simulink model "processor_with_peripherals"  (R2025a)
settings: Solver=FixedStepDiscrete  StartTime=0.0  StopTime=inf  RelTol=1e-3
libraries: simulink x6
(part 2 of 5)

== system processor_with_peripherals/Processor ==
  In1 : Inport
  Common hardware : Subsystem
  Core_0 : Subsystem
  Core_1 : Subsystem
  Core_2 : Subsystem
  Core_3 : Subsystem
  Instruction_Memory_{0..3} (4 alike) : LookupNDDirect  NumberOfTableDimensions=1  Table=[808464698;808464432;926496560;1144140337;1144402484;1145123890;1128608816;1144401989;1127362614;892810038;221463092;808532490;808529968;808464432;892874808;959460404;959985974;858798390;876098866;825771568;1144469044;1162098229;825887245;842018864;909127728;1110454339;909193785;960639283;825241653;943009843;842023737;826356273;859125811;973737267;808464433;808464435;843266352;1093810480;926167618;925906232;910378291;892351281;1160982584;808470085;168637495;808464698;808465456;909130032;1111049269;926496582;1144140337;1144402484;1145123890;1128608816;1144401989;221852470;808532490;808792112;926101552;808466741;892874808;959985972;959460406;858797110;959984946;1144473136;893662773;825887245;909127728;909127728;925904963;1160983097;859975987;826689077;943011891;1160921908;825766449;892678195;973737271;808464433;808464439;843265072;942815555;927089732;825307444;909390128;892612921;892614962;910374448;168641336;808464698;808466480;842610480;892813878;942682167;1093874224;808927555;1128542533;909719609;875640885;221458999;808532490;809054256;959459376;825767732;858863156;808465968;859385905;892613944;858862659;808465712;927281200;825887245;1093677104;1160785968;1144008774;943140912;943011385;808924209;943141941;825635889;808857651;959459632;973737272;808464433;808464450;892875577;893596976;892351281;875573300;808470085;909127733;808470085;926036034;168638278;808464698;808469296;1093742640;926103344;859058224;1093742640;926103344;859058224;1093742640;808927792;221328951;808532490;809775152;842018864;1127821364;825504564;892350769;1160984372;843200067;927086388;842020656;875966516;825887245;1160785968;959459376;876036920;942747697;909129778;808662323;825372725;1177892659;1095118901;859255876;973737264;808464433;808464454;1160852278;808465734;925906754;808727088;859063097;860041529;1178745155;925906754;168636721;808464698;808464433;875638832;876099888;876823607;909325875;808928819;1094267696;942815288;808923952;221398071;808532490;808530224;825241648;858927156;925904946;826421296;858928950;925905970;859385904;925906744;943273267;825887245;842084400;892350512;942883651;825701444;942883651;875575346;808530225;1110852406;808923191;1144009777;973737285;825241649;808464435;926168368;927152196;808470085;959590457;826489137;808465207;808464432;808727106;168641605;808464698;808465457;808530992;942815281;808923952;875573303;875771952;808792119;1160853808;942815283;221790512;808532490;808792368;892350512;1127298352;893662019;825771586;859191092;910570289;842543152;858992696;842217272;825887245;909193264;1177563184;942682165;808858675;858796087;1178021939;942682165;842477621;1144008755;825241655;973737269;825241649;808464439;927085893;909721906;926433601;859386678;808466243;808989240;925906232;1178088257;168637751;808464698;808466481;1178026544;1110787141;808663366;808794167;893663024;1128478007;1127756081;1128478005;221786421;808532490;809054512;1127297072;858929475;892350514;842543152;858927160;892352562;842543152;876163128;959459636;825887245;1093742640;1177563184;825701700;943140915;909127733;1178876211;825241654;1144599619;1144206392;875643704;973737284;825241649;808464450;927154992;893600569;860046147;825508657;960706616;925906232;826491697;808989240;168637238;808464698;808469297;943800880;876098871;875573555;1177765171;1177961284;1111769925;875836727;876097841;221660469;808532490;809775408;1127297072;943274292;875902531;876884803;859190068;910242617;943992880;943272771;1127297844;825887245;1160851504;842018864;808989235;925904949;959918404;942883640;942879800;925906994;808466227;1160786740;973737283;825241649;808464454;925906754;808988720;1144338480;927019832;808466228;892547889;808465713;860174649;168636977;808464698;808464434;909326128;859058224;942815280;825308208;1128346673;942814000;875574073;1127625265;221591346;808532490;808530480;875573296;842155061;909128771;1093809731;892351544;1127297605;1144533300;942686789;875640116;825887245;842149936;1160785968;825241670;843134768;808727091;942682164;808726581;1111704628;842019890 ...(+53136 chars)]
  Scope : Scope
      settings: ActiveDisplayYMinimum=-5.4492107336360064E+9  ActiveDisplayYMaximum=2.1970867278297868E+9  DataLoggingVariableName=ScopeData8
  Address : Outport
  MemWrite : Outport  Port=2
  RAM_WData : Outport  Port=3
  wires:
  Core_3/2(Out2) -> Common hardware/1(In1)
  Core_1/2(Out2) -> Core_2/2(In2)
  Instruction_Memory_2/1 -> Core_2/1(In1)
  Core_2/2(Out2) -> Core_3/2(In2)
  Common hardware/1(Out1) -> Core_0/1(In1)
  Instruction_Memory_3/1 -> Core_3/1(In1)
  Core_3/1(Out1) -> Instruction_Memory_3/1
  Core_2/1(Out1) -> Instruction_Memory_2/1
  Instruction_Memory_0/1 -> Scope/1, Core_0/2(In2)
  Core_1/1(Out1) -> Instruction_Memory_1/1
  Core_0/2(Out2) -> Core_1/1(In2)
  Core_0/1(Out1) -> Instruction_Memory_0/1
  Instruction_Memory_1/1 -> Core_1/2(In1)
  Common hardware/2(Out2) -> MemWrite/1
  Common hardware/3(Out3) -> Address/1
  Common hardware/4(RAM_WData) -> RAM_WData/1
  In1/1 -> Common hardware/2(In2)
